simulink model "plutoradioFrequencyCorrectionRx"  (R2023a)
settings: Solver=FixedStepDiscrete  StartTime=0.0  StopTime=62.91456  RelTol=1e-3  EnableMultiTasking=on
undefined symbols (not defined in the file or in its folder): Fs, ip, usb
libraries: plutoradiolib x1
settings Model: Creator=The MathWorks, Inc.  LastModifiedBy=The MathWorks, Inc.
settings SolverCC: AlgebraicLoopSolver=TrustRegion
settings DataIOCC: LimitDataPoints=on  SaveFormat=Array  ReturnWorkspaceOutputs=off
settings OptimizationCC: ExpressionDepthLimit=2147483647  LifeSpan=inf
settings DebuggingCC: UnderspecifiedInitializationDetection=Classic  MergeDetectMultiDrivingBlocksExec=none  SolverPrmCheckMsg=warning  ParameterPrecisionLossMsg=none  FcnCallInpInsideContextMsg=warning  UnconnectedInputMsg=warning  UnconnectedOutputMsg=warning  UnconnectedLineMsg=warning  AllowSymbolicDim=off  StateNameClashWarn=warning  SFUnexpectedBacktrackingDiag=warning  SFNoUnconditionalDefaultTransitionDiag=warning  SFExecutionAtInitializationDiag=none  ArithmeticOperatorsInVariantConditions=warning
settings HardwareCC: ProdBitPerPointer=32  ProdBitPerSizeT=32  ProdBitPerPtrDiffT=32  ProdLargestAtomicFloat=None  ProdIntDivRoundTo=Undefined  ProdEndianess=Unspecified  ProdWordSize=32  ProdHWDeviceType=32-bit Generic  TargetBitPerLong=64  TargetBitPerPointer=64  TargetBitPerSizeT=64  TargetBitPerPtrDiffT=64  TargetLongLongMode=on  TargetIntDivRoundTo=Zero  TargetEndianess=LittleEndian  TargetWordSize=64  TargetHWDeviceType=Generic->MATLAB Host Computer  ProdEqTarget=off
settings ModelReferenceCC: EnableRefExpFcnMdlSchedulingChecks=on  PropagateSignalLabelsOutOfModel=off
settings SFSimCC: SimUseLocalCustomCode=off  CustomCodeUndefinedFunction=UseInterfaceOnly
settings RTWCC: RTWUseLocalCustomCode=off
settings RTWCC: CustomSourceCode=|
  | #include<stdio.h>
  | #include<stdlib.h>
settings CodeAppCC: StateflowObjectComments=on
settings GRTTargetCC: TargetLangStandard=C89/C90 (ANSI)  CombineOutputUpdateFcns=off  GRTInterface=on
settings ConfigComp: CovMetricSettings=dw  CovSaveCumulativeToWorkspaceVar=on  CovSaveSingleToWorkspaceVar=on  CovExternalEMLEnable=off  CovSFcnEnable=off

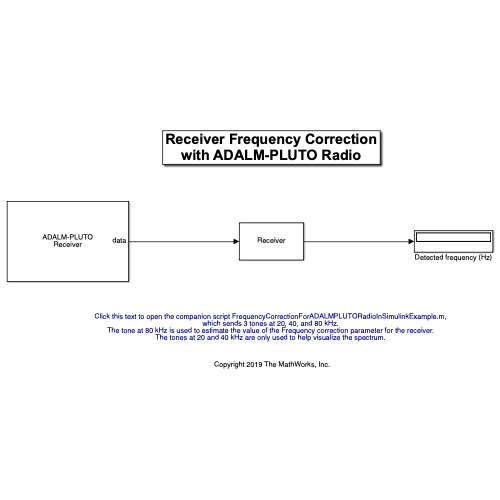
[thumbnail: Simulink's stored preview of the top-level diagram]
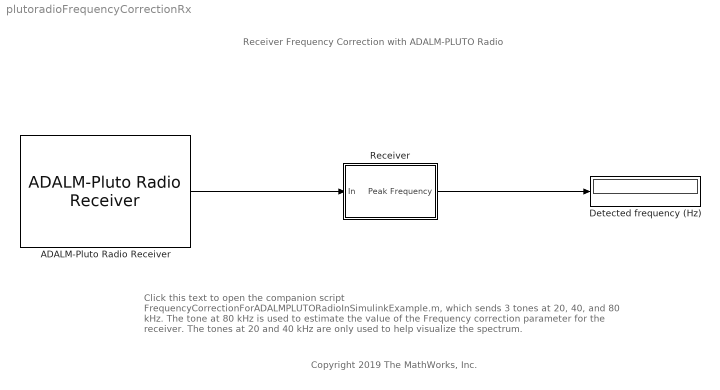
== system plutoradioFrequencyCorrectionRx ==
  note: Receiver Frequency Correction
      | with ADALM-PLUTO Radio
  note: Click this text to open the companion script FrequencyCorrectionForADALMPLUTORadioInSimulinkExample.m,
      | which sends 3 tones at 20, 40, and 80 kHz.
      | The tone at 80 kHz is used to estimate the value of the Frequency correction parameter for the receiver.
      | The tones at 20 and 40 kHz are only used to help visualize the spectrum.
  note: Copyright 2019 The MathWorks, Inc.
  ADALM-Pluto Radio Receiver : plutoradiolib/ADALM-Pluto Radio Receiver  RadioID=usb:0  uri=ip:10.0.0.200  CenterFrequencySource=Dialog  CenterFrequency=2.42e9  GainSource=AGC Fast Attack  GainSourceBlock=AGC Slow Attack  Gain=20  ChannelMapping=1  BasebandSampleRate=200e3  OutputDataType=double  SamplesPerFrame=1024*1024  OverflowOutputPort=off  EnableBurstMode=off  NumFramesInBurst=1  ShowAdvancedProperties=off  UseCustomFilter=off  filtPathRates=[737280000 11520000 3840000 1920000 960000 240000]  filtCoefficients=[-192 82 85 -215 228 -102 -110 290 -318 145 160 -426 471 -215 -238 633 -697 318 349 -923 1009 -457 -498 1309 -1423 640 693 -1812 1959 -876 -945 2458 -2647 1180 1268 -3290 3534 -1572 -1688 4375 -4698 2091 2247 -5836 6284 -2807 -3031 7918 -8588 3870 4225 -11182 12324 -5662 -6330 17255 -19735 9507 11312 -33568 43355 -25227 -42139 305542 305542 -42139 -25227 43355 -33568 11312 9507 -19735 17255 -6330 -5662 12324 -11182 4225 3870 -8588 7918 -3031 -2807 6284 -5836 2247 2091 -4698 4375 -1688 -1572 3534 -3290 1268 1180 -2647 2458 -945 -876 1959 -1812 693 640 -1423 1309 -498 -457 1009 -923 349 318 -697 633 -238 -215 471 -426 160 145 -318 290 -110 -102 228 -215 85 82 -192]  filtCoefficientSize=128  filtDecimInterpFactor=4  filtGain=-12  filtRFBandwidth=18000000  filterConfigStruct=struct()  EnableQuadratureCorrection=on  EnableRFDCCorrection=on  EnableBasebandDCCorrection=on  FrequencyCorrection=0  OverrideSampleTime=off  SampleTime=0.02  DataTimeout=Inf  ENSMPinControlMode=None  BISTLoopbackMode=Disabled  BISTToneInject=Disabled  BISTSignalGen=PRBS  BISTToneFreq=Fs/32  BISTToneLevel=0
  Detected frequency (Hz) : Display
  Receiver : Subsystem
      mask Display: disp('Receiver')
  wires:
  Receiver/1("Peak Frequency ") -> Detected frequency (Hz)/1
  ADALM-Pluto Radio Receiver/1 -> Receiver/1(In)

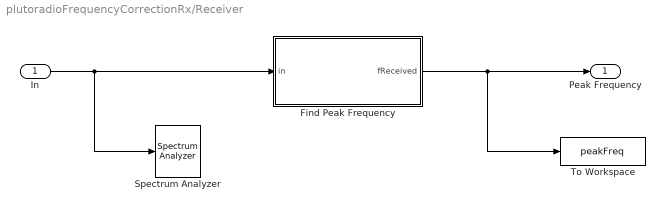
== system plutoradioFrequencyCorrectionRx/Receiver ==
  In : Inport
  Find Peak Frequency : MATLAB Function  TreatAsAtomicUnit=on
  Spectrum Analyzer : SpectrumAnalyzer  WindowPosition=[30 503 933 509]  Method=Welch  SampleRate=200000  Span=200000  StartFrequency=-100000  StopFrequency=100000  AveragingMethod=Running  YLimits=[-110.10796417087610166,29.138856518603283519]  DefaultConfigurationName=spbscopes.SpectrumAnalyzerBlockCfg  IsFrequencyInputMode=0  FrequencyVectorPort=0  FrequencyVectorFromPort=0  FrequencyInputRBWPort=0  FrequencyInputRBWFromPort=0
  To Workspace : ToWorkspace  VariableName=peakFreq  SampleTime=-1
      settings: MaxDataPoints=1
  "Peak Frequency " : Outport  VectorParamsAs1DForOutWhenUnconnected=off
  wires:
  Find Peak Frequency/1(fReceived) -> To Workspace/1, "Peak Frequency "/1
  In/1 -> Find Peak Frequency/1(in), Spectrum Analyzer/1

== matlab function plutoradioFrequencyCorrectionRx/Receiver/Find Peak Frequency ==
  data: fReceived output; in input
function fReceived  = findpeakfreq(in)
% Find the frequency of the received tone corresponding to the 80 kHz
% tone transmitted by plutoradioFrequencyCorrectionSimulinkExample.m

%#codegen

FFTSig = fftshift(abs(fft(in)));
FFTSize = length(FFTSig);

% plutoradioFrequencyCorrectionSimulinkExample.m sends 3 tones
% at 20, 40, and 80 kHz

[~, idx] = findpeaks(FFTSig,'MinPeakProminence',max(0.5*FFTSig));
fReceived = (max(idx)-FFTSize/2-1)/FFTSize*200e3;
